simulink model "check_Differential"  (R2018b)
settings: configuration reference "Physics" (kept outside this file)
model workspace (MAT data in the model file):
  veh_param = Simulink.Parameter
  veh_param.Value.cLiftF = 0
  veh_param.Value.cLiftR = 0
  veh_param.Value.CoGx_m = 0
  veh_param.Value.CoGy_m = 0
  veh_param.Value.CoGz_m = 0
  veh_param.Value.cDrag = 0
  veh_param.Value.Aref_m2 = 0
  veh_param.Value.Gearratio = 0
  veh_param.Value.Wheelbase_m = 0
  veh_param.Value.PacLatF = [0 0 0 0 0]
  veh_param.Value.PacLongF = [0 0 0 0 0]
  veh_param.Value.PacLatR = [0 0 0 0 0]
  veh_param.Value.PacLongR = [0 0 0 0 0]
  veh_param.Value.cRollFriction_Npmps = 0
  veh_param.Value.MaxRollFriction_N = 0
  veh_param.Value.T_YawRate_s = 0
  veh_param.Value.T_LatVel_s = 0
  veh_param.Value.TrackWidthF_m = 0
  veh_param.Value.TrackWidthR_m = 0
  veh_param.Value.TireRadiusF_m = 0
  veh_param.Value.TireRadiusR_m = 0
  veh_param.Value.VehicleInertia_kgm2 = 0
  veh_param.Value.WheelInertiaF_kgm2 = 0
  veh_param.Value.WheelInertiaR_kgm2 = 0
  veh_param.Value.VehicleMass_kg = 0
  veh_param.Value.switchModelBlend_mps = 0
  veh_param.Value.PTLimitLowVel_N = 0
  veh_param.Value.switchModelVel_mps = 0
  veh_param.Value.T_Tire_s = 0
  veh_param.DataType = 'struct'
  veh_param.Dimensions = [1 1]
  x0_positionstates = Simulink.Parameter
  x0_positionstates.Value = [0 0 0]
  x0_positionstates.DataType = 'auto'
  x0_positionstates.Dimensions = [1 3]
undefined symbols (not defined in the file): POWTR__DIFFERENTIAL__c_diff_efficiency, POWTR__DIFFERENTIAL__c_diff_ratio, POWTR__DIFFERENTIAL__f_diff_efficiency, POWTR__DIFFERENTIAL__f_diff_ratio, POWTR__DIFFERENTIAL__r_diff_efficiency, POWTR__DIFFERENTIAL__r_diff_ratio, POWTR__LAYOUT__p_torque_rear, tireFL__MFSIMPLE__r_tire_m, tireFR__MFSIMPLE__r_tire_m, tireRL__MFSIMPLE__r_tire_m, tireRR__MFSIMPLE__r_tire_m, VEH__VehicleData__l_WheelbaseF_m, VEH__VehicleData__l_WheelbaseTotal_m, VEH__VehicleData__w_TrackF_m, VEH__VehicleData__w_TrackR_m
settings Model: DataDictionary=vehicleparameters_vehdynsim.sldd  OrderedModelArguments=off  Creator=wischnewski  LastModifiedBy=ga25xiw

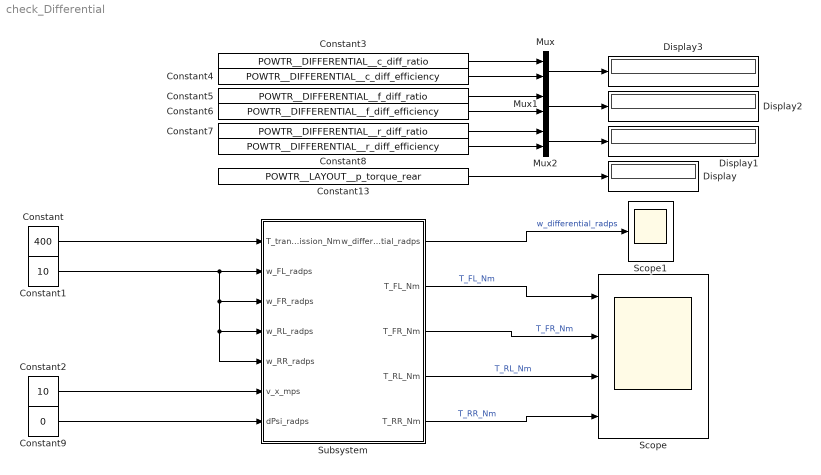
== system check_Differential ==
  Constant : Constant  Value=400
  Constant1 : Constant  Value=10
  Constant13 : Constant  Value=POWTR__LAYOUT__p_torque_rear
  Constant2 : Constant  Value=10
  Constant3 : Constant  Value=POWTR__DIFFERENTIAL__c_diff_ratio
  Constant4 : Constant  Value=POWTR__DIFFERENTIAL__c_diff_efficiency
  Constant5 : Constant  Value=POWTR__DIFFERENTIAL__f_diff_ratio
  Constant6 : Constant  Value=POWTR__DIFFERENTIAL__f_diff_efficiency
  Constant7 : Constant  Value=POWTR__DIFFERENTIAL__r_diff_ratio
  Constant8 : Constant  Value=POWTR__DIFFERENTIAL__r_diff_efficiency
  Constant9 : Constant  Value=0
  Display{,1..3} (4 alike) : Display
  Mux : Mux  Inputs=2
  Mux1 : Mux  Inputs=2
  Mux2 : Mux  Inputs=2
  Scope : Scope  NumInputPorts=4
  Scope1 : Scope
  Subsystem : Subsystem
  wires:
  Constant/1 -> Subsystem/1(T_transmission_Nm)
  Constant1/1 -> Subsystem/2(w_FL_radps), Subsystem/3(w_FR_radps), Subsystem/4(w_RL_radps), Subsystem/5(w_RR_radps)
  Constant13/1 -> Display/1
  Constant8/1 -> Mux2/2
  Constant7/1 -> Mux2/1
  Constant5/1 -> Mux1/1
  Constant3/1 -> Mux/1
  Constant6/1 -> Mux1/2
  Constant4/1 -> Mux/2
  Mux/1 -> Display3/1
  Mux1/1 -> Display2/1
  Mux2/1 -> Display1/1
  Subsystem/5(T_RR_Nm) -> Scope/4  "T_RR_Nm"
  Subsystem/4(T_RL_Nm) -> Scope/3  "T_RL_Nm"
  Subsystem/3(T_FR_Nm) -> Scope/2  "T_FR_Nm"
  Subsystem/2(T_FL_Nm) -> Scope/1  "T_FL_Nm"
  Subsystem/1(w_differential_radps) -> Scope1/1  "w_differential_radps"
  Constant2/1 -> Subsystem/6(v_x_mps)
  Constant9/1 -> Subsystem/7(dPsi_radps)

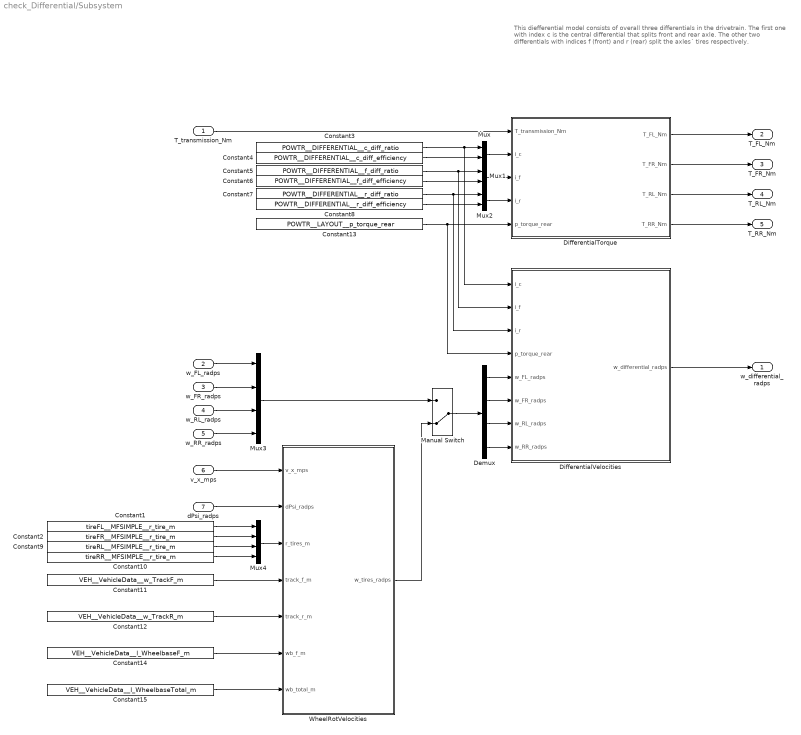
== system check_Differential/Subsystem ==
  note: This diefferential model consists of overall three differentials in the drivetrain.
      | The first one with index c is the central differential that splits front and rear axle.
      | The other two differentials with indices f (front) and r (rear) split the axles´ tires respectively.
  T_transmission_Nm : Inport
  w_FL_radps : Inport  Port=2
  w_FR_radps : Inport  Port=3
  w_RL_radps : Inport  Port=4
  w_RR_radps : Inport  Port=5
  v_x_mps : Inport  Port=6
  dPsi_radps : Inport  Port=7
  Constant1 : Constant  Value=tireFL__MFSIMPLE__r_tire_m
  Constant10 : Constant  Value=tireRR__MFSIMPLE__r_tire_m
  Constant11 : Constant  Value=VEH__VehicleData__w_TrackF_m
  Constant12 : Constant  Value=VEH__VehicleData__w_TrackR_m
  Constant13 : Constant  Value=POWTR__LAYOUT__p_torque_rear
  Constant14 : Constant  Value=VEH__VehicleData__l_WheelbaseF_m
  Constant15 : Constant  Value=VEH__VehicleData__l_WheelbaseTotal_m
  Constant2 : Constant  Value=tireFR__MFSIMPLE__r_tire_m
  Constant3 : Constant  Value=POWTR__DIFFERENTIAL__c_diff_ratio
  Constant4 : Constant  Value=POWTR__DIFFERENTIAL__c_diff_efficiency
  Constant5 : Constant  Value=POWTR__DIFFERENTIAL__f_diff_ratio
  Constant6 : Constant  Value=POWTR__DIFFERENTIAL__f_diff_efficiency
  Constant7 : Constant  Value=POWTR__DIFFERENTIAL__r_diff_ratio
  Constant8 : Constant  Value=POWTR__DIFFERENTIAL__r_diff_efficiency
  Constant9 : Constant  Value=tireRL__MFSIMPLE__r_tire_m
  Demux : Demux
  DifferentialTorque : MATLAB Function  TreatAsAtomicUnit=on
  DifferentialVelocities : MATLAB Function  TreatAsAtomicUnit=on
  Manual Switch : ManualSwitch  CurrentSetting=0
  Mux : Mux  Inputs=2
  Mux1 : Mux  Inputs=2
  Mux2 : Mux  Inputs=2
  Mux3 : Mux
  Mux4 : Mux
  WheelRotVelocities : MATLAB Function  TreatAsAtomicUnit=on
  w_differential_radps : Outport
  T_FL_Nm : Outport  Port=2
  T_FR_Nm : Outport  Port=3
  T_RL_Nm : Outport  Port=4
  T_RR_Nm : Outport  Port=5
  wires:
  Constant12/1 -> WheelRotVelocities/5(track_r_m)
  Mux4/1 -> WheelRotVelocities/3(r_tires_m)
  Constant15/1 -> WheelRotVelocities/7(wb_total_m)
  DifferentialVelocities/1(w_differential_radps) -> w_differential_radps/1
  Constant3/1 -> Mux/1, DifferentialVelocities/1(i_c)
  Mux3/1 -> Manual Switch/1
  Manual Switch/1 -> Demux/1
  Constant1/1 -> Mux4/1
  Demux/2 -> DifferentialVelocities/6(w_FR_radps)
  Demux/3 -> DifferentialVelocities/7(w_RL_radps)
  Constant9/1 -> Mux4/3
  Constant10/1 -> Mux4/4
  Demux/1 -> DifferentialVelocities/5(w_FL_radps)
  Mux1/1 -> DifferentialTorque/3(i_f)
  Constant4/1 -> Mux/2
  WheelRotVelocities/1(w_tires_radps) -> Manual Switch/2
  T_transmission_Nm/1 -> DifferentialTorque/1(T_transmission_Nm)
  DifferentialTorque/1(T_FL_Nm) -> T_FL_Nm/1
  Constant11/1 -> WheelRotVelocities/4(track_f_m)
  Constant5/1 -> Mux1/1, DifferentialVelocities/2(i_f)
  w_FR_radps/1 -> Mux3/2
  dPsi_radps/1 -> WheelRotVelocities/2(dPsi_radps)
  Demux/4 -> DifferentialVelocities/8(w_RR_radps)
  Constant13/1 -> DifferentialTorque/5(p_torque_rear), DifferentialVelocities/4(p_torque_rear)
  DifferentialTorque/3(T_RL_Nm) -> T_RL_Nm/1
  w_RL_radps/1 -> Mux3/3
  DifferentialTorque/2(T_FR_Nm) -> T_FR_Nm/1
  Constant7/1 -> Mux2/1, DifferentialVelocities/3(i_r)
  v_x_mps/1 -> WheelRotVelocities/1(v_x_mps)
  w_RR_radps/1 -> Mux3/4
  Constant2/1 -> Mux4/2
  Constant14/1 -> WheelRotVelocities/6(wb_f_m)
  Constant8/1 -> Mux2/2
  Mux2/1 -> DifferentialTorque/4(i_r)
  w_FL_radps/1 -> Mux3/1
  Constant6/1 -> Mux1/2
  DifferentialTorque/4(T_RR_Nm) -> T_RR_Nm/1
  Mux/1 -> DifferentialTorque/2(i_c)

== matlab function check_Differential/Subsystem/DifferentialTorque ==
  data: T_transmission_Nm input; i_c input; T_FL_Nm output; i_f input; i_r input; p_torque_rear input; T_FR_Nm output; T_RL_Nm output; T_RR_Nm output
function [T_FL_Nm, T_FR_Nm, T_RL_Nm, T_RR_Nm] = fcn(...
                        T_transmission_Nm, i_c, i_f, i_r, p_torque_rear)

[T_FL_Nm, T_FR_Nm, T_RL_Nm, T_RR_Nm] = DifferentialTorque(...
                        T_transmission_Nm, i_c, i_f, i_r, p_torque_rear);

== matlab function check_Differential/Subsystem/DifferentialVelocities ==
  data: i_c input; w_differential_radps output; i_f input; i_r input; p_torque_rear input; w_FL_radps input; w_FR_radps input; w_RL_radps input; w_RR_radps input
function w_differential_radps = fcn(...
                        i_c, i_f, i_r, p_torque_rear, ...
                        w_FL_radps, w_FR_radps, w_RL_radps, w_RR_radps)

w_differential_radps = DifferentialVelocities(...
                        i_c, i_f, i_r, p_torque_rear, ...
                        w_FL_radps, w_FR_radps, w_RL_radps, w_RR_radps);

== matlab function check_Differential/Subsystem/WheelRotVelocities ==
  data: v_x_mps input; w_tires_radps output; dPsi_radps input; r_tires_m input; track_f_m input; track_r_m input; wb_f_m input; wb_total_m input
function w_tires_radps = fcn(v_x_mps, dPsi_radps, r_tires_m, ...
            track_f_m, track_r_m, wb_f_m, wb_total_m)

w_tires_radps = WheelRotVelocities(v_x_mps, dPsi_radps, r_tires_m, ...
            track_f_m, track_r_m, wb_f_m, wb_total_m);
